simulink model "sim_Baseline_Claw"  (Simulink 7.2)
settings: Solver=ode5  StartTime=0.0  StopTime=tsim  FixedStep=ts  RelTol=1e-3
undefined symbols (not defined in the file or in its folder): CA, fc, invCB, ka, Kb, kq, Ma, Md, Mq, stepcmd, tcmd, Za, Zd
settings Model: Creator=E183308  LastModifiedBy=E183308
settings DataIOCC: SaveOutput=off  SignalLogging=off  SaveTime=off
settings OptimizationCC: InitFltsAndDblsToZero=on
settings DebuggingCC: SaveWithParameterizedLinksMsg=none  SignalResolutionControl=TryResolveAllWithWarning  MultiTaskDSMMsg=warning  MultiTaskCondExecSysMsg=none
settings RTWCC: IncludeERTFirstTime=on
settings GRTTargetCC: TargetFcnLib=ansi_tfl_tmw.mat

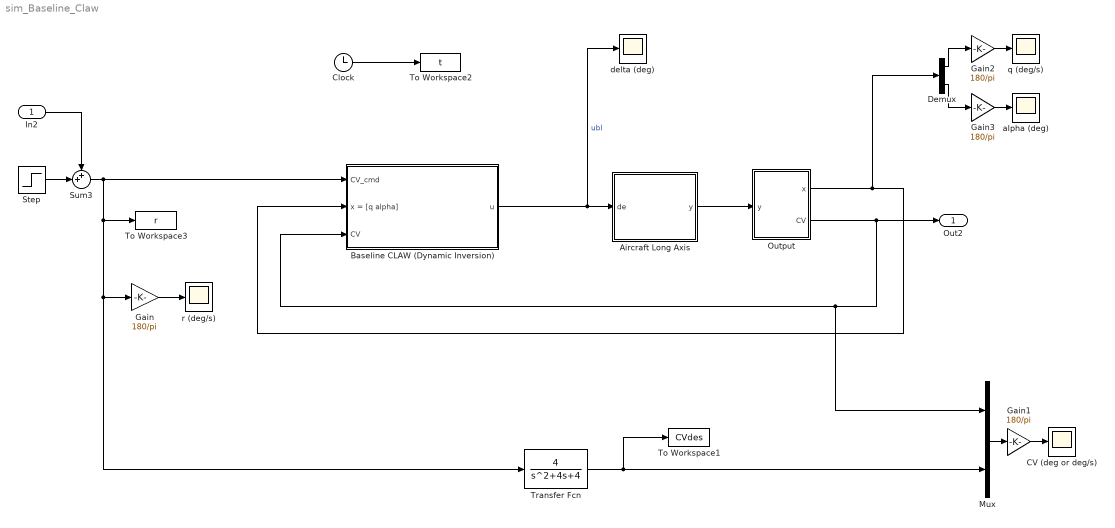
== system sim_Baseline_Claw ==
  In2 : Inport  OutDataType=sfix(16)  OutScaling=2^0
  Aircraft Long Axis : Subsystem
  Baseline CLAW (Dynamic Inversion) : Subsystem
  CV (deg or deg/s) : Scope
      settings: TimeRange=15  YMin=0  YMax=12
  Clock : Clock
      settings: Decimation=10
  Demux : Demux  Outputs=2
  Gain{,1..3} (4 alike) : Gain  Gain=180/pi  ParameterDataType=sfix(16)  ParameterScaling=2^0  OutDataType=sfix(16)  OutScaling=2^0
  Mux : Mux  Inputs=2
  Output : Subsystem
  Step : Step  Time=tcmd  After=stepcmd  SampleTime=0
  Sum3 : Sum  Inputs=++|  OutDataType=sfix(16)  OutScaling=2^0
  To Workspace1 : ToWorkspace  VariableName=CVdes  SampleTime=-1  SaveFormat=Array
  To Workspace2 : ToWorkspace  VariableName=t  SampleTime=-1  SaveFormat=Array
  To Workspace3 : ToWorkspace  VariableName=r  SampleTime=-1  SaveFormat=Array
  Transfer Fcn : TransferFcn  Numerator=4  Denominator=[1 4 4]
  alpha (deg) : Scope
      settings: TimeRange=20  YMin=0  YMax=14  SaveName=ScopeData5
  delta (deg) : Scope
      settings: TimeRange=20  YMin=-20  YMax=10  SaveName=ScopeData6
  q (deg/s) : Scope
      settings: TimeRange=20  YMin=0  SaveName=ScopeData4
  r (deg/s) : Scope
      settings: TimeRange=40  SaveName=ScopeData8
  Out2 : Outport  OutDataType=sfix(16)  OutScaling=2^0
  wires:
  Step/1 -> Sum3/2
  Sum3/1 -> To Workspace3/1, Gain/1, Transfer Fcn/1, Baseline CLAW (Dynamic Inversion)/1(CV_cmd)
  Baseline CLAW (Dynamic Inversion)/1(u) -> delta (deg)/1, Aircraft Long Axis/1(de)  "ubl"
  Output/2(CV) -> Out2/1, Mux/1, Baseline CLAW (Dynamic Inversion)/3(CV)
  Output/1(x) -> Demux/1, Baseline CLAW (Dynamic Inversion)/2(x = [q alpha])
  In2/1 -> Sum3/1
  Gain/1 -> r (deg/s)/1
  Mux/1 -> Gain1/1
  Gain1/1 -> CV (deg or deg/s)/1
  Gain2/1 -> q (deg/s)/1
  Gain3/1 -> alpha (deg)/1
  Demux/1 -> Gain2/1
  Demux/2 -> Gain3/1
  Transfer Fcn/1 -> Mux/2, To Workspace1/1
  Aircraft Long Axis/1(y) -> Output/1(y)
  Clock/1 -> To Workspace2/1

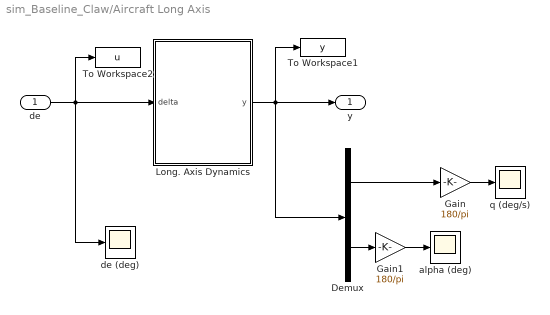
== system sim_Baseline_Claw/Aircraft Long Axis ==
  de : Inport  OutDataType=sfix(16)  OutScaling=2^0
  Demux : Demux  Outputs=[1 1]
  Gain : Gain  Gain=180/pi  ParameterDataType=sfix(16)  ParameterScaling=2^0  OutDataType=sfix(16)  OutScaling=2^0
  Gain1 : Gain  Gain=180/pi  ParameterDataType=sfix(16)  ParameterScaling=2^0  OutDataType=sfix(16)  OutScaling=2^0
  Long. Axis Dynamics : Subsystem
  To Workspace1 : ToWorkspace  VariableName=y  SampleTime=-1  SaveFormat=Array
  To Workspace2 : ToWorkspace  VariableName=u  SampleTime=-1  SaveFormat=Array
  alpha (deg) : Scope
      settings: TimeRange=10  YMin=0  SaveName=ScopeData10
  de (deg) : Scope
      settings: TimeRange=10  YMin=-20  YMax=20  SaveName=ScopeData3
  q (deg/s) : Scope
      settings: TimeRange=10  YMin=0  SaveName=ScopeData2
  y : Outport  OutDataType=sfix(16)  OutScaling=2^0
  wires:
  Demux/1 -> Gain/1
  Demux/2 -> Gain1/1
  Gain1/1 -> alpha (deg)/1
  de/1 -> To Workspace2/1, de (deg)/1, Long. Axis Dynamics/1(delta)
  Gain/1 -> q (deg/s)/1
  Long. Axis Dynamics/1(y) -> Demux/1, y/1, To Workspace1/1

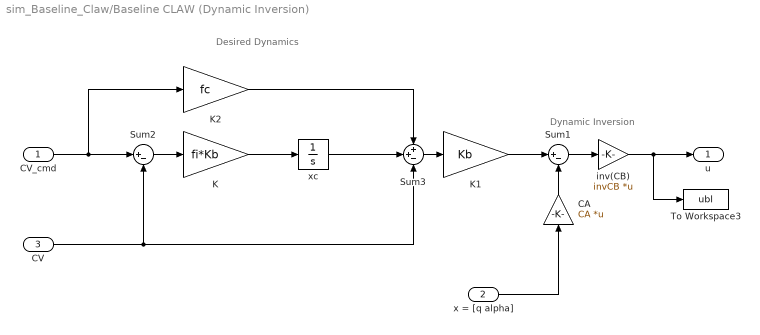
== system sim_Baseline_Claw/Baseline CLAW (Dynamic Inversion) ==
  note: Desired
      | Dynamics
  note: Dynamic
      | Inversion
  CV_cmd : Inport  OutDataType=sfix(16)  OutScaling=2^0
  x = [q alpha] : Inport  Port=2  OutDataType=sfix(16)  OutScaling=2^0
  CV : Inport  Port=3  OutDataType=sfix(16)  OutScaling=2^0
  CA : Gain  Orientation=up  Gain=CA  Multiplication=Matrix(K*u)  ParameterDataType=sfix(16)  ParameterScaling=2^0  OutDataType=sfix(16)  OutScaling=2^0
  K : Gain  Gain=fi*Kb  ParameterDataType=sfix(16)  ParameterScaling=2^0  OutDataType=sfix(16)  OutScaling=2^0
  K1 : Gain  Gain=Kb  ParameterDataType=sfix(16)  ParameterScaling=2^0  OutDataType=sfix(16)  OutScaling=2^0
  K2 : Gain  Gain=fc  ParameterDataType=sfix(16)  ParameterScaling=2^0  OutDataType=sfix(16)  OutScaling=2^0
  Sum1 : Sum  Inputs=|+-  OutDataType=sfix(16)  OutScaling=2^0
  Sum2 : Sum  Inputs=|+-  OutDataType=sfix(16)  OutScaling=2^0
  Sum3 : Sum  Inputs=++-  OutDataType=sfix(16)  OutScaling=2^0
  To Workspace3 : ToWorkspace  VariableName=ubl  SampleTime=-1  SaveFormat=Array
  inv(CB) : Gain  Gain=invCB  Multiplication=Matrix(K*u)  ParameterDataType=sfix(16)  ParameterScaling=2^0  OutDataType=sfix(16)  OutScaling=2^0
  xc : Integrator
  u : Outport  OutDataType=sfix(16)  OutScaling=2^0
  wires:
  Sum1/1 -> inv(CB)/1
  CA/1 -> Sum1/2
  CV_cmd/1 -> Sum2/1, K2/1
  inv(CB)/1 -> u/1, To Workspace3/1
  x = [q alpha]/1 -> CA/1
  K/1 -> xc/1
  Sum2/1 -> K/1
  xc/1 -> Sum3/2
  CV/1 -> Sum2/2, Sum3/3
  Sum3/1 -> K1/1
  K2/1 -> Sum3/1
  K1/1 -> Sum1/1

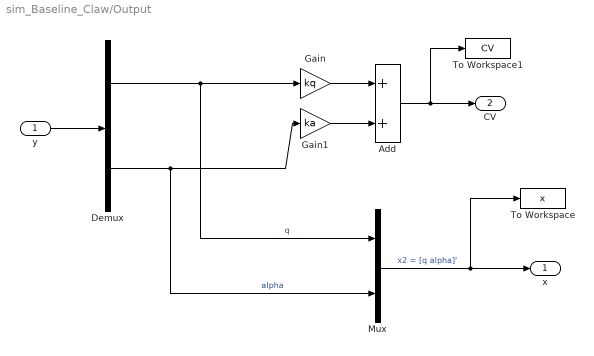
== system sim_Baseline_Claw/Output ==
  y : Inport  OutDataType=sfix(16)  OutScaling=2^0
  Add : Sum  OutDataType=sfix(16)  OutScaling=2^-10
  Demux : Demux  Outputs=[1 1]
  Gain : Gain  Gain=kq  ParameterDataType=sfix(16)  ParameterScaling=2^0  OutDataType=sfix(16)  OutScaling=2^0
  Gain1 : Gain  Gain=ka  ParameterDataType=sfix(16)  ParameterScaling=2^0  OutDataType=sfix(16)  OutScaling=2^0
  Mux : Mux  Inputs=[1 1]
  To Workspace : ToWorkspace  VariableName=x  SampleTime=-1  SaveFormat=Array
  To Workspace1 : ToWorkspace  VariableName=CV  SampleTime=-1  SaveFormat=Array
  x : Outport  OutDataType=sfix(16)  OutScaling=2^0
  CV : Outport  Port=2  OutDataType=sfix(16)  OutScaling=2^0
  wires:
  Demux/2 -> Mux/2, Gain1/1  "alpha"
  Demux/1 -> Mux/1, Gain/1  "q"
  Add/1 -> To Workspace1/1, CV/1
  Gain1/1 -> Add/2
  Gain/1 -> Add/1
  y/1 -> Demux/1
  Mux/1 -> To Workspace/1, x/1  "x2 = [q alpha]'"

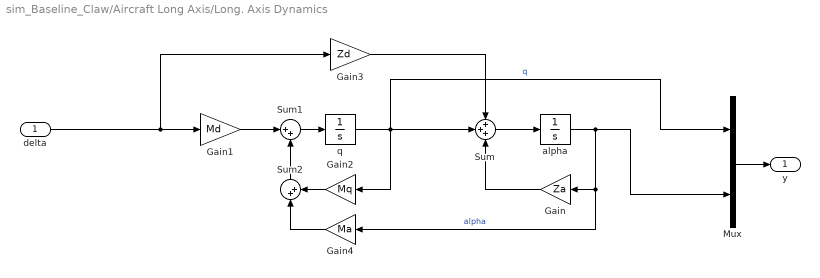
== system sim_Baseline_Claw/Aircraft Long Axis/Long. Axis Dynamics ==
  delta : Inport  OutDataType=sfix(16)  OutScaling=2^0
  Gain : Gain  Orientation=left  Gain=Za  ParameterDataType=sfix(16)  ParameterScaling=2^0  OutDataType=sfix(16)  OutScaling=2^0  SaturateOnIntegerOverflow=on  OutDataTypeStr=Inherit: Same as input  ParamDataTypeStr=Inherit: Same as input
  Gain1 : Gain  Gain=Md  ParameterDataType=sfix(16)  ParameterScaling=2^0  OutDataType=sfix(16)  OutScaling=2^0  SaturateOnIntegerOverflow=on  OutDataTypeStr=Inherit: Same as input  ParamDataTypeStr=Inherit: Same as input
  Gain2 : Gain  Orientation=left  Gain=Mq  ParameterDataType=sfix(16)  ParameterScaling=2^0  OutDataType=sfix(16)  OutScaling=2^0  SaturateOnIntegerOverflow=on  OutDataTypeStr=Inherit: Same as input  ParamDataTypeStr=Inherit: Same as input
  Gain3 : Gain  Gain=Zd  ParameterDataType=sfix(16)  ParameterScaling=2^0  OutDataType=sfix(16)  OutScaling=2^0  SaturateOnIntegerOverflow=on  OutDataTypeStr=Inherit: Same as input  ParamDataTypeStr=Inherit: Same as input
  Gain4 : Gain  Orientation=left  Gain=Ma  ParameterDataType=sfix(16)  ParameterScaling=2^0  OutDataType=sfix(16)  OutScaling=2^0  SaturateOnIntegerOverflow=on  OutDataTypeStr=Inherit: Same as input  ParamDataTypeStr=Inherit: Same as input
  Mux : Mux  Inputs=2
  Sum : Sum  Inputs=+++  OutDataType=sfix(16)  OutScaling=2^0  SaturateOnIntegerOverflow=on  InputSameDT=on  OutDataTypeStr=Inherit: Same as first input
  Sum1 : Sum  Inputs=|++  OutDataType=sfix(16)  OutScaling=2^0  SaturateOnIntegerOverflow=on  InputSameDT=on  OutDataTypeStr=Inherit: Same as first input
  Sum2 : Sum  Orientation=up  Inputs=|++  OutDataType=sfix(16)  OutScaling=2^0  SaturateOnIntegerOverflow=on  InputSameDT=on  OutDataTypeStr=Inherit: Same as first input
  alpha : Integrator
  q : Integrator
  y : Outport  OutDataType=sfix(16)  OutScaling=2^0
  wires:
  delta/1 -> Gain3/1, Gain1/1
  q/1 -> Sum/2, Mux/1, Gain2/1  "q"
  Gain/1 -> Sum/3
  Sum/1 -> alpha/1
  alpha/1 -> Mux/2, Gain4/1, Gain/1  "alpha"
  Sum1/1 -> q/1
  Gain1/1 -> Sum1/1
  Gain3/1 -> Sum/1
  Gain2/1 -> Sum2/2
  Sum2/1 -> Sum1/2
  Gain4/1 -> Sum2/1
  Mux/1 -> y/1
